simulink model "ModeStatCtrl"  (R2018b)
settings: Solver=FixedStepDiscrete  StartTime=0.0  StopTime=10.0  FixedStep=0.01  RelTol=1e-3
settings Model: Creator=sn2xws  LastModifiedBy=sn2xws
settings ModelReferenceCC: ModelReferenceNumInstancesAllowed=Single

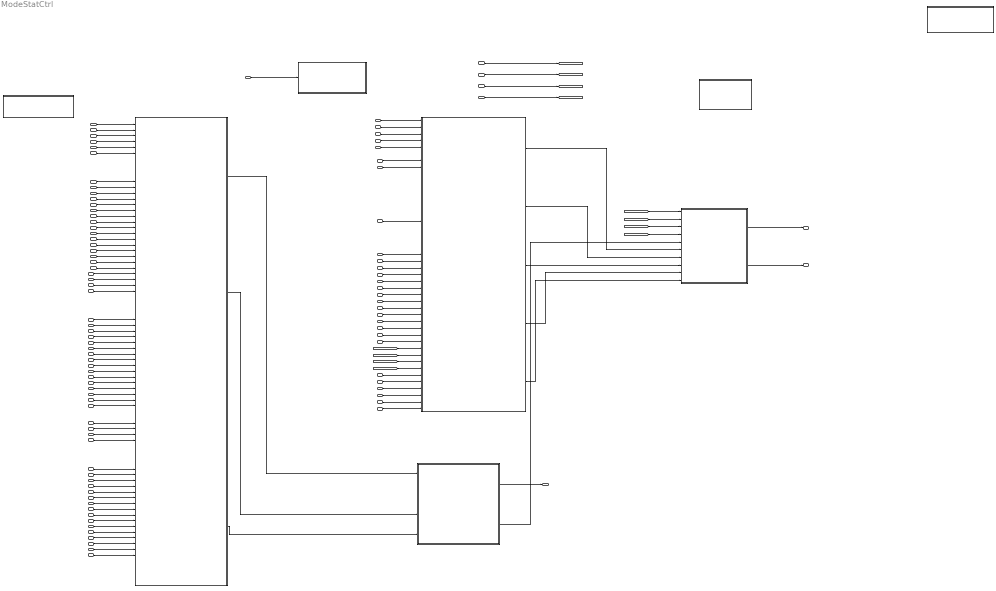
== system ModeStatCtrl ==
  CommCond_Val : Inport  OutDataTypeStr=boolean  PortDimensions=1
  CommExitCond_Val : Inport  Port=2  OutDataTypeStr=boolean  PortDimensions=1
  CommExitCondwithSpeed_Val : Inport  Port=3  OutDataTypeStr=boolean  PortDimensions=1
  SoftIntAcsEnty_Val : Inport  Port=4  OutDataTypeStr=IntEnable  PortDimensions=1
  SoftIntAcsExt_Val : Inport  Port=5  OutDataTypeStr=IntEnable  PortDimensions=1
  SoftIntAllLug_Val : Inport  Port=6  OutDataTypeStr=IntEnable  PortDimensions=1
  SoftIntAllVip_Val : Inport  Port=7  OutDataTypeStr=IntEnable  PortDimensions=1
  SoftIntIntimacyRt_Val : Inport  Port=8  OutDataTypeStr=IntEnable  PortDimensions=1
  SoftIntINTM_Val : Inport  Port=9  OutDataTypeStr=IntEnable  PortDimensions=1
  SoftIntLfFamly_Val : Inport  Port=10  OutDataTypeStr=IntEnable  PortDimensions=1
  SoftIntLfLug_Val : Inport  Port=11  OutDataTypeStr=IntEnable  PortDimensions=1
  SoftIntLfLy_Val : Inport  Port=12  OutDataTypeStr=IntEnable  PortDimensions=1
  SoftIntLfRcvy_Val : Inport  Port=13  OutDataTypeStr=IntEnable  PortDimensions=1
  SoftIntLfVip_Val : Inport  Port=14  OutDataTypeStr=IntEnable  PortDimensions=1
  SoftIntLgrstCloseLt_Val : Inport  Port=15  OutDataTypeStr=IntEnable  PortDimensions=1
  SoftIntLgrstCloseRt_Val : Inport  Port=16  OutDataTypeStr=IntEnable  PortDimensions=1
  SoftIntLgrstOpenLt_Val : Inport  Port=17  OutDataTypeStr=IntEnable  PortDimensions=1
  SoftIntLgrstOpenRt_Val : Inport  Port=18  OutDataTypeStr=IntEnable  PortDimensions=1
  SoftIntRtFamly_Val : Inport  Port=19  OutDataTypeStr=IntEnable  PortDimensions=1
  SoftIntRtLug_Val : Inport  Port=20  OutDataTypeStr=IntEnable  PortDimensions=1
  SoftIntRtLy_Val : Inport  Port=21  OutDataTypeStr=IntEnable  PortDimensions=1
  SoftIntRtRcvy_Val : Inport  Port=22  OutDataTypeStr=IntEnable  PortDimensions=1
  SoftIntRtVip_Val : Inport  Port=23  OutDataTypeStr=IntEnable  PortDimensions=1
  SwIntAcsEnty_Val : Inport  Port=24  OutDataTypeStr=IntEnable  PortDimensions=1
  SwIntAcsExt_Val : Inport  Port=25  OutDataTypeStr=IntEnable  PortDimensions=1
  SwIntAllLug_Val : Inport  Port=26  OutDataTypeStr=IntEnable  PortDimensions=1
  SwIntAllVip_Val : Inport  Port=27  OutDataTypeStr=IntEnable  PortDimensions=1
  SwIntIntimacyRt_Val : Inport  Port=28  OutDataTypeStr=IntEnable  PortDimensions=1
  SwIntINTM_Val : Inport  Port=29  OutDataTypeStr=IntEnable  PortDimensions=1
  SwIntLfFamly_Val : Inport  Port=30  OutDataTypeStr=IntEnable  PortDimensions=1
  SwIntLfLug_Val : Inport  Port=31  OutDataTypeStr=IntEnable  PortDimensions=1
  SwIntLfLy_Val : Inport  Port=32  OutDataTypeStr=IntEnable  PortDimensions=1
  SwIntLfRcvy_Val : Inport  Port=33  OutDataTypeStr=IntEnable  PortDimensions=1
  SwIntLfVip_Val : Inport  Port=34  OutDataTypeStr=IntEnable  PortDimensions=1
  SwIntLgrstCloseLt_Val : Inport  Port=35  OutDataTypeStr=IntEnable  PortDimensions=1
  SwIntLgrstCloseRt_Val : Inport  Port=36  OutDataTypeStr=IntEnable  PortDimensions=1
  SwIntLgrstOpenLt_Val : Inport  Port=37  OutDataTypeStr=IntEnable  PortDimensions=1
  SwIntLgrstOpenRt_Val : Inport  Port=38  OutDataTypeStr=IntEnable  PortDimensions=1
  SwIntRtFamly_Val : Inport  Port=39  OutDataTypeStr=IntEnable  PortDimensions=1
  SwIntRtLug_Val : Inport  Port=40  OutDataTypeStr=IntEnable  PortDimensions=1
  SwIntRtLy_Val : Inport  Port=41  OutDataTypeStr=IntEnable  PortDimensions=1
  SwIntRtRcvy_Val : Inport  Port=42  OutDataTypeStr=IntEnable  PortDimensions=1
  SwIntRtVip_Val : Inport  Port=43  OutDataTypeStr=IntEnable  PortDimensions=1
  acsEntyMdReq_Val : Inport  Port=44  OutDataTypeStr=boolean  PortDimensions=1
  acsExtMdReq_Val : Inport  Port=45  OutDataTypeStr=boolean  PortDimensions=1
  AllLugMdReq_Val : Inport  Port=46  OutDataTypeStr=boolean  PortDimensions=1
  AllVipMdReq_Val : Inport  Port=47  OutDataTypeStr=boolean  PortDimensions=1
  IntimacyRtMdReq_Val : Inport  Port=48  OutDataTypeStr=boolean  PortDimensions=1
  INTMMdReq_Val : Inport  Port=49  OutDataTypeStr=boolean  PortDimensions=1
  LfFamlyReq_Val : Inport  Port=50  OutDataTypeStr=boolean  PortDimensions=1
  LfLyMdReq_Val : Inport  Port=51  OutDataTypeStr=boolean  PortDimensions=1
  LgrstCloseLtMdReq_Val : Inport  Port=52  OutDataTypeStr=boolean  PortDimensions=1
  LgrstCloseRtMdReq_Val : Inport  Port=53  OutDataTypeStr=boolean  PortDimensions=1
  LgrstOpenLtMdReq_Val : Inport  Port=54  OutDataTypeStr=boolean  PortDimensions=1
  LgrstOpenRtMdReq_Val : Inport  Port=55  OutDataTypeStr=boolean  PortDimensions=1
  LtLugMdReq_Val : Inport  Port=56  OutDataTypeStr=boolean  PortDimensions=1
  LtRcvyMdReq_Val : Inport  Port=57  OutDataTypeStr=boolean  PortDimensions=1
  LtVipMdReq_Val : Inport  Port=58  OutDataTypeStr=boolean  PortDimensions=1
  RtFamlyMdReq_Val : Inport  Port=59  OutDataTypeStr=boolean  PortDimensions=1
  RtLugMdReq_Val : Inport  Port=60  OutDataTypeStr=boolean  PortDimensions=1
  RtLyMdReq_Val : Inport  Port=61  OutDataTypeStr=boolean  PortDimensions=1
  RtRcvyMdReq_Val : Inport  Port=62  OutDataTypeStr=boolean  PortDimensions=1
  RtVipMdReq_Val : Inport  Port=63  OutDataTypeStr=boolean  PortDimensions=1
  LugMdLtAvl_Val : Inport  Port=64  OutDataTypeStr=boolean  PortDimensions=1
  LugMdRtAvl_Val : Inport  Port=65  OutDataTypeStr=boolean  PortDimensions=1
  VipMdLtAvl_Val : Inport  Port=66  OutDataTypeStr=boolean  PortDimensions=1
  VipMdRtAvl_Val : Inport  Port=67  OutDataTypeStr=boolean  PortDimensions=1
  acsEntyMdSrcTp_Val : Inport  Port=68  OutDataTypeStr=Enum: SrcReqTp1  PortDimensions=1
  acsExtMdSrcTp_Val : Inport  Port=69  OutDataTypeStr=Enum: SrcReqTp1  PortDimensions=1
  AllLugSrcReqTp_Val : Inport  Port=70  OutDataTypeStr=Enum: SrcReqTp1  PortDimensions=1
  AllVipSrcReqTp_Val : Inport  Port=71  OutDataTypeStr=Enum: SrcReqTp1  PortDimensions=1
  IntimacyRtMdSrcTp_Val : Inport  Port=72  OutDataTypeStr=Enum: SrcReqTp1  PortDimensions=1
  INTMSrcReqTp_Val : Inport  Port=73  OutDataTypeStr=Enum: SrcReqTp1  PortDimensions=1
  LfFamlySrcReqTp_Val : Inport  Port=74  OutDataTypeStr=Enum: SrcReqTp1  PortDimensions=1
  LfLySrcReqTp_Val : Inport  Port=75  OutDataTypeStr=Enum: SrcReqTp1  PortDimensions=1
  LgrstCloseLtSrcReqTp_Val : Inport  Port=76  OutDataTypeStr=Enum: SrcReqTp1  PortDimensions=1
  LgrstCloseRtSrcReqTp_Val : Inport  Port=77  OutDataTypeStr=Enum: SrcReqTp1  PortDimensions=1
  LgrstOpenLtSrcReqTp_Val : Inport  Port=78  OutDataTypeStr=Enum: SrcReqTp1  PortDimensions=1
  LgrstOpenRtSrcReqTp_Val : Inport  Port=79  OutDataTypeStr=Enum: SrcReqTp1  PortDimensions=1
  LtLugSrcReqTp_Val : Inport  Port=80  OutDataTypeStr=Enum: SrcReqTp1  PortDimensions=1
  LtRcvySrcReqTp_Val : Inport  Port=81  OutDataTypeStr=Enum: SrcReqTp1  PortDimensions=1
  LtVipSrcReqTp_Val : Inport  Port=82  OutDataTypeStr=Enum: SrcReqTp1  PortDimensions=1
  RtFamlySrcReqTp_Val : Inport  Port=83  OutDataTypeStr=Enum: SrcReqTp1  PortDimensions=1
  RtLugSrcReqTp_Val : Inport  Port=84  OutDataTypeStr=Enum: SrcReqTp1  PortDimensions=1
  RtLySrcReqTp_Val : Inport  Port=85  OutDataTypeStr=Enum: SrcReqTp1  PortDimensions=1
  RtRcvySrcReqTp_Val : Inport  Port=86  OutDataTypeStr=Enum: SrcReqTp1  PortDimensions=1
  RtVipSrcReqTp_Val : Inport  Port=87  OutDataTypeStr=Enum: SrcReqTp1  PortDimensions=1
  WelcomeBkwdMdReq : Inport  Port=88  OutDataTypeStr=boolean  PortDimensions=1
  WelcomeFwdMdReq : Inport  Port=89  OutDataTypeStr=boolean  PortDimensions=1
  SecRwLtStFwdBkwdPos : Inport  Port=90  OutDataTypeStr=uint16  PortDimensions=1
  SecRwRtStFwdBkwdPos : Inport  Port=91  OutDataTypeStr=uint16  PortDimensions=1
  StNumFlg_Is4s : Inport  Port=92
  StNumFlg_Is6s : Inport  Port=93
  StNumFlg_Is6s7s : Inport  Port=94
  StNumFlg_Is7s : Inport  Port=95
  MdEnCtrlAndBsyChk : Subsystem
  Model : ModelReference  ModelNameDialog=StateOnOffChk.slx  SimulationMode=Normal  ModelReferenceVersion=V2.0.0
  Model1 : ModelReference  ModelNameDialog=MdXX_QuitReason.slx  SimulationMode=Normal  ModelReferenceVersion=V2.0.0
  Model2 : ModelReference  ModelNameDialog=MdSWReqChk.slx  SimulationMode=Normal  ModelReferenceVersion=V2.0.0
  Model3 : ModelReference  ModelNameDialog=MdXXArray.slx  SimulationMode=Normal  ModelReferenceVersion=V2.0.0
  Model4 : ModelReference  ModelNameDialog=ModeStateCtrlCaller.slx  SimulationMode=Normal  ModelReferenceVersion=V2.0.0
  Model6 : ModelReference  ModelNameDialog=MdXX_QuitChk.slx  SimulationMode=Normal  ModelReferenceVersion=V2.0.0
  Model7 : ModelReference  ModelNameDialog=ModeStatAndRspCallerForTest.slx  SimulationMode=Normal  ModelReferenceVersion=V2.0.0
  MdXX_QuitArray : Outport  OutDataTypeStr=Enum: MdRspLocal2  PortDimensions=32
  modestate32_Val : Outport  Port=2  OutDataTypeStr=uint32  PortDimensions=1
  IsStBsy32Bit_Val : Outport  Port=3  OutDataTypeStr=uint32  PortDimensions=1
  wires:
  CommExitCond_Val/1 -> Model3/5
  CommExitCondwithSpeed_Val/1 -> Model3/6
  Model6/1 -> MdXX_QuitArray/1
  MdEnCtrlAndBsyChk/2(IsStBsy32Bit_Val) -> IsStBsy32Bit_Val/1
  acsEntyMdSrcTp_Val/1 -> Model3/1
  acsExtMdSrcTp_Val/1 -> Model3/2
  AllLugSrcReqTp_Val/1 -> Model3/3
  AllVipSrcReqTp_Val/1 -> Model3/4
  IntimacyRtMdSrcTp_Val/1 -> Model3/11
  INTMSrcReqTp_Val/1 -> Model3/12
  LfFamlySrcReqTp_Val/1 -> Model3/13
  LfLySrcReqTp_Val/1 -> Model3/14
  LgrstCloseLtSrcReqTp_Val/1 -> Model3/15
  LgrstCloseRtSrcReqTp_Val/1 -> Model3/16
  LgrstOpenLtSrcReqTp_Val/1 -> Model3/17
  LgrstOpenRtSrcReqTp_Val/1 -> Model3/18
  LtLugSrcReqTp_Val/1 -> Model3/19
  LtRcvySrcReqTp_Val/1 -> Model3/20
  LtVipSrcReqTp_Val/1 -> Model3/21
  RtLugSrcReqTp_Val/1 -> Model3/23
  RtLySrcReqTp_Val/1 -> Model3/24
  RtRcvySrcReqTp_Val/1 -> Model3/25
  RtVipSrcReqTp_Val/1 -> Model3/26
  CommCond_Val/1 -> Model/1
  StNumFlg_Is4s/1 -> [StNumFlg_Is4s]
  StNumFlg_Is6s/1 -> [StNumFlg_Is6s]
  StNumFlg_Is6s7s/1 -> [StNumFlg_Is6s7s]
  StNumFlg_Is7s/1 -> [StNumFlg_Is7s]
  SoftIntAcsEnty_Val/1 -> Model3/27
  SoftIntAcsExt_Val/1 -> Model3/28
  SoftIntAllLug_Val/1 -> Model3/29
  SoftIntAllVip_Val/1 -> Model3/30
  SoftIntIntimacyRt_Val/1 -> Model3/35
  SoftIntINTM_Val/1 -> Model3/36
  SoftIntLfFamly_Val/1 -> Model3/37
  SoftIntLfLug_Val/1 -> Model3/38
  SoftIntLfLy_Val/1 -> Model3/39
  SoftIntLfRcvy_Val/1 -> Model3/40
  SoftIntLfVip_Val/1 -> Model3/41
  SoftIntLgrstCloseLt_Val/1 -> Model3/42
  SoftIntLgrstCloseRt_Val/1 -> Model3/43
  SoftIntLgrstOpenLt_Val/1 -> Model3/44
  SoftIntLgrstOpenRt_Val/1 -> Model3/45
  SoftIntRtLug_Val/1 -> Model3/47
  SoftIntRtFamly_Val/1 -> Model3/46
  SoftIntRtLy_Val/1 -> Model3/48
  SoftIntRtRcvy_Val/1 -> Model3/49
  SoftIntRtVip_Val/1 -> Model3/50
  acsEntyMdReq_Val/1 -> Model2/1
  acsExtMdReq_Val/1 -> Model2/2
  AllLugMdReq_Val/1 -> Model2/3
  LtRcvyMdReq_Val/1 -> Model2/4
  LtVipMdReq_Val/1 -> Model2/5
  RtRcvyMdReq_Val/1 -> Model2/7
  RtVipMdReq_Val/1 -> Model2/8
  AllVipMdReq_Val/1 -> Model2/16
  IntimacyRtMdReq_Val/1 -> Model2/21
  INTMMdReq_Val/1 -> Model2/22
  LfFamlyReq_Val/1 -> Model2/23
  LfLyMdReq_Val/1 -> Model2/24
  LgrstCloseLtMdReq_Val/1 -> Model2/25
  LgrstCloseRtMdReq_Val/1 -> Model2/26
  LgrstOpenLtMdReq_Val/1 -> Model2/27
  LgrstOpenRtMdReq_Val/1 -> Model2/28
  LtLugMdReq_Val/1 -> Model2/29
  LugMdLtAvl_Val/1 -> Model2/30
  LugMdRtAvl_Val/1 -> Model2/31
  RtFamlyMdReq_Val/1 -> Model2/32
  RtLugMdReq_Val/1 -> Model2/33
  RtLyMdReq_Val/1 -> Model2/34
  VipMdLtAvl_Val/1 -> Model2/39
  VipMdRtAvl_Val/1 -> Model2/40
  [StNumFlg_Is4s] -> Model2/35
  [StNumFlg_Is6s] -> Model2/36
  [StNumFlg_Is6s7s] -> Model2/37
  [StNumFlg_Is7s] -> Model2/38
  Model3/1 -> Model6/1
  Model3/2 -> Model6/3
  Model3/4 -> Model6/4
  SwIntAcsEnty_Val/1 -> Model3/53
  SwIntAcsExt_Val/1 -> Model3/54
  SwIntAllLug_Val/1 -> Model3/55
  SwIntAllVip_Val/1 -> Model3/56
  SwIntIntimacyRt_Val/1 -> Model3/61
  SwIntINTM_Val/1 -> Model3/62
  SwIntLfFamly_Val/1 -> Model3/63
  SwIntLfLug_Val/1 -> Model3/64
  SwIntLfLy_Val/1 -> Model3/65
  SwIntLfRcvy_Val/1 -> Model3/66
  SwIntLfVip_Val/1 -> Model3/67
  SwIntLgrstCloseLt_Val/1 -> Model3/68
  SwIntLgrstCloseRt_Val/1 -> Model3/69
  SwIntLgrstOpenLt_Val/1 -> Model3/70
  SwIntLgrstOpenRt_Val/1 -> Model3/71
  SwIntRtFamly_Val/1 -> Model3/72
  SwIntRtLug_Val/1 -> Model3/73
  SwIntRtLy_Val/1 -> Model3/74
  SwIntRtRcvy_Val/1 -> Model3/75
  SwIntRtVip_Val/1 -> Model3/76
  [StNumFlg_Is7s] -> MdEnCtrlAndBsyChk/4(StNumFlg_Is7s)
  [StNumFlg_Is6s7s] -> MdEnCtrlAndBsyChk/3(StNumFlg_Is6s7s)
  [StNumFlg_Is6s] -> MdEnCtrlAndBsyChk/2(StNumFlg_Is6s)
  [StNumFlg_Is4s] -> MdEnCtrlAndBsyChk/1(StNumFlg_Is4s)
  Model2/1 -> MdEnCtrlAndBsyChk/6(ChkBsyBitArray)
  Model2/2 -> MdEnCtrlAndBsyChk/7(MdReqArray)
  Model2/3 -> MdEnCtrlAndBsyChk/8(SetBsyBitArray)
  Model2/4 -> MdEnCtrlAndBsyChk/9(SetEnBitArray)
  Model2/5 -> MdEnCtrlAndBsyChk/10(VeSMSuMdNum)
  Model6/2 -> MdEnCtrlAndBsyChk/5(MdXX_Quit32Bit_Val)
  MdEnCtrlAndBsyChk/1(modestate32_Val) -> modestate32_Val/1
  RtFamlySrcReqTp_Val/1 -> Model3/22
  WelcomeBkwdMdReq/1 -> Model2/41
  WelcomeFwdMdReq/1 -> Model2/42
  SecRwLtStFwdBkwdPos/1 -> Model2/43
  SecRwRtStFwdBkwdPos/1 -> Model2/44

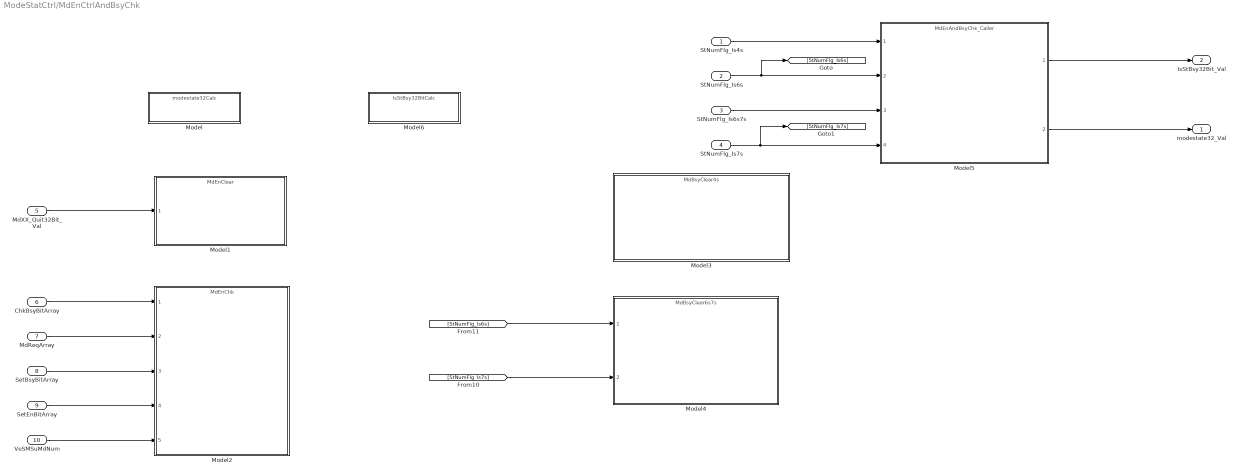
== system ModeStatCtrl/MdEnCtrlAndBsyChk ==
  StNumFlg_Is4s : Inport
  StNumFlg_Is6s : Inport  Port=2
  StNumFlg_Is6s7s : Inport  Port=3
  StNumFlg_Is7s : Inport  Port=4
  MdXX_Quit32Bit_Val : Inport  Port=5
  ChkBsyBitArray : Inport  Port=6
  MdReqArray : Inport  Port=7
  SetBsyBitArray : Inport  Port=8
  SetEnBitArray : Inport  Port=9
  VeSMSuMdNum : Inport  Port=10
  Model : ModelReference  ModelNameDialog=modestate32Calc.slx  SimulationMode=Normal  ModelReferenceVersion=V2.0.0
  Model1 : ModelReference  ModelNameDialog=MdEnClear.slx  SimulationMode=Normal  ModelReferenceVersion=V2.0.0
  Model2 : ModelReference  ModelNameDialog=MdEnChk.slx  SimulationMode=Normal  ModelReferenceVersion=V2.0.0
  Model3 : ModelReference  ModelNameDialog=MdBsyClear4s.slx  SimulationMode=Normal  ModelReferenceVersion=V2.0.0
  Model4 : ModelReference  ModelNameDialog=MdBsyClear6s7s.slx  SimulationMode=Normal  ModelReferenceVersion=V2.0.0
  Model5 : ModelReference  ModelNameDialog=MdEnAndBsyChk_Caller.slx  SimulationMode=Normal  ModelReferenceVersion=V2.0.0
  Model6 : ModelReference  ModelNameDialog=IsStBsy32BitCalc.slx  SimulationMode=Normal  ModelReferenceVersion=V2.0.0
  modestate32_Val : Outport  OutDataTypeStr=uint32  PortDimensions=1
  IsStBsy32Bit_Val : Outport  Port=2  OutDataTypeStr=uint32  PortDimensions=1
  wires:
  StNumFlg_Is6s/1 -> [StNumFlg_Is6s], Model5/2
  StNumFlg_Is4s/1 -> Model5/1
  StNumFlg_Is6s7s/1 -> Model5/3
  StNumFlg_Is7s/1 -> [StNumFlg_Is7s], Model5/4
  [StNumFlg_Is6s] -> Model4/1
  [StNumFlg_Is7s] -> Model4/2
  MdXX_Quit32Bit_Val/1 -> Model1/1
  ChkBsyBitArray/1 -> Model2/1
  MdReqArray/1 -> Model2/2
  SetBsyBitArray/1 -> Model2/3
  SetEnBitArray/1 -> Model2/4
  VeSMSuMdNum/1 -> Model2/5
  Model5/2 -> modestate32_Val/1
  Model5/1 -> IsStBsy32Bit_Val/1
